simulink model "GravitationalBattery"  (R2020b)
settings: Solver=VariableStepAuto  StartTime=0.0  StopTime=1000000  RelTol=1e-9  AbsTol=1e-9
model workspace (MAT data in the model file):
  Sig = Simulink.Signal
  Sig.DataType = 'auto'
  Sig.Dimensions = -1
  Sig.DimensionsMode = 'auto'
  Sig.Complexity = 'auto'
  Sig.SampleTime = -1
  Sig.SamplingMode = 'auto'
  Sig1 = Simulink.Signal
  Sig1.DataType = 'auto'
  Sig1.Dimensions = -1
  Sig1.DimensionsMode = 'auto'
  Sig1.Complexity = 'auto'
  Sig1.SampleTime = -1
  Sig1.SamplingMode = 'auto'
  Sig2 = Simulink.Signal
  Sig2.DataType = 'auto'
  Sig2.Dimensions = -1
  Sig2.DimensionsMode = 'auto'
  Sig2.Complexity = 'auto'
  Sig2.SampleTime = -1
  Sig2.SamplingMode = 'auto'
  earth_gravitational_acceleration = Simulink.Parameter
  earth_gravitational_acceleration.Value = -9.806
  earth_gravitational_acceleration.Description = 'https://en.wikipedia.org/wiki/Standard_gravity'
  earth_gravitational_acceleration.DataType = 'double'
  earth_gravitational_acceleration.DocUnits = 'm^2/s'
  earth_gravitational_acceleration.Dimensions = [1 1]
  electrogenerator_coeff = Simulink.Parameter
  electrogenerator_coeff.DataType = 'double'
  electrogenerator_coeff.Min = 0
  electrogenerator_coeff.DocUnits = 'V/(rad/s)'
  electrogenerator_coeff.Dimensions = [0 0]
  gear_box_ration = Simulink.Parameter
  gear_box_ration.Value = 1
  gear_box_ration.Description = 'Gear box ration'
  gear_box_ration.DataType = 'double'
  gear_box_ration.Min = 0
  gear_box_ration.Dimensions = [1 1]
  initial_mass_height = Simulink.Parameter
  initial_mass_height.Value = 10000
  initial_mass_height.Description = 'https://en.wikipedia.org/wiki/Distance'
  initial_mass_height.DataType = 'double'
  initial_mass_height.Min = 0
  initial_mass_height.DocUnits = 'm'
  initial_mass_height.Dimensions = [1 1]
  resistance_value = Simulink.Parameter
  resistance_value.Value = 1
  resistance_value.Description = 'https://en.wikipedia.org/wiki/Electrical_resistance_and_conductance'
  resistance_value.DataType = 'double'
  resistance_value.Min = 0
  resistance_value.DocUnits = 'Ohm'
  resistance_value.Dimensions = [1 1]
  weight_mass = Simulink.Parameter
  weight_mass.Value = 1
  weight_mass.Description = 'https://en.wikipedia.org/wiki/Mass'
  weight_mass.DataType = 'double'
  weight_mass.Min = 0
  weight_mass.DocUnits = 'kg'
  weight_mass.Dimensions = [1 1]
  wheel_and_axel_radius = Simulink.Parameter
  wheel_and_axel_radius.Value = 1
  wheel_and_axel_radius.Description = 'Radius of perfect wheel and axel mechanism'
  wheel_and_axel_radius.DataType = 'double'
  wheel_and_axel_radius.Min = 0
  wheel_and_axel_radius.DocUnits = 'm'
  wheel_and_axel_radius.Dimensions = [1 1]
libraries: fl_lib x15, nesl_utility x9, simulink x1, sdl_lib x1
Description:
  | https://en.wikipedia.org/wiki/Gravity_battery
settings Model: OrderedModelArguments=off  Creator=ofcra  LastModifiedBy=ofcra
settings SolverCC: InitialStep=1

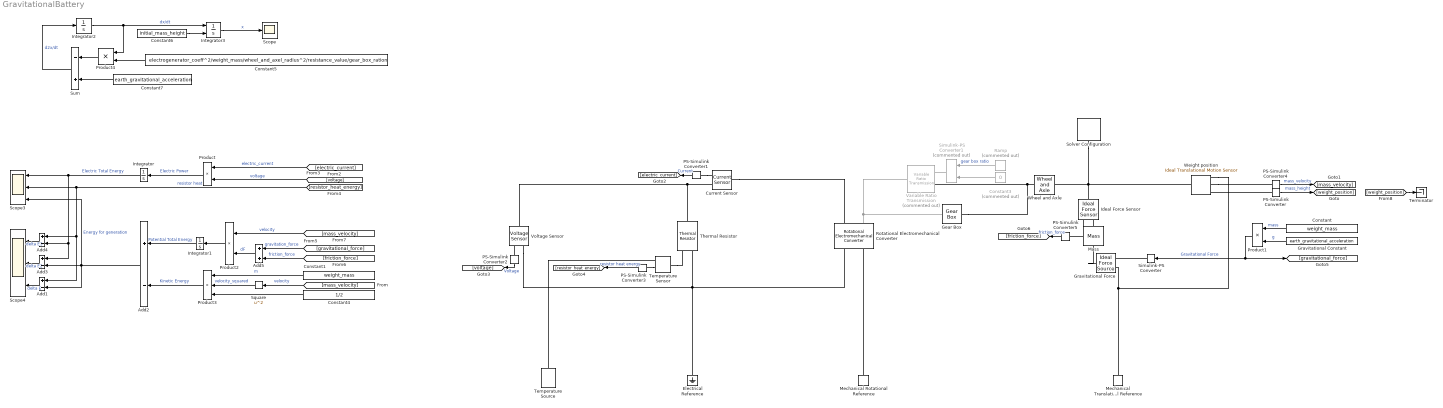
== system GravitationalBattery ==
  Add{1..4} (4 alike) : Sum  Inputs=+-
  Add5 : Sum
  Constant : Constant  Value=weight_mass
  Constant1 : Constant  Value=weight_mass
  Constant3 : Constant  Commented=on  Value=0
  Constant4 : Constant  Value=1/2
  Constant5 : Constant  Value=electrogenerator_coeff^2/weight_mass/wheel_and_axel_radius^2/resistance_value/gear_box_ration
  Constant6 : Constant  Value=initial_mass_height
  Constant7 : Constant  Value=earth_gravitational_acceleration
  Current Sensor : fl_lib/Electrical/Electrical Sensors/Current Sensor
  Electrical Reference : fl_lib/Electrical/Electrical Elements/Electrical Reference
  Gear Box : fl_lib/Mechanical/Mechanisms/Gear Box  ratio=gear_box_ration  t_in_specify=off  t_in_priority=None  t_in=0 N*m  t_in_nominal_specify=off  t_in_nominal_unit=N*m  t_in_nominal_value=1  t_out_specify=off  t_out_priority=None  t_out=0 N*m  t_out_nominal_specify=off  t_out_nominal_unit=N*m  t_out_nominal_value=1
  Gravitational Constant : Constant  Value=earth_gravitational_acceleration
  Gravitational Force : fl_lib/Mechanical/Mechanical Sources/Ideal Force Source
  Ideal Force Sensor : fl_lib/Mechanical/Mechanical Sensors/Ideal Force Sensor
  Integrator : Integrator
  Integrator1 : Integrator
  Integrator2 : Integrator
  Integrator3 : Integrator  InitialConditionSource=external
  Mass : fl_lib/Mechanical/Translational Elements/Mass  mass=weight_mass kg  num_ports=foundation.enum.numPorts2.two  v_specify=off  v_priority=High  v=0 m/s  v_nominal_specify=off  v_nominal_unit=m/s  v_nominal_value=1  f_specify=off  f_priority=None  f=0 N  f_nominal_specify=off  f_nominal_unit=N  f_nominal_value=1
      settings: InternalSimscapePortConfiguration="{\"Bottom\":[],\"Left\":[{\"id\":\"M\",\"label\":\"\",\"type\":\"foundation.mechanical.translational.translational\"}],\"Right\":[{\"id\":\"N\",\"label\":\"\",\"type\":\"foundation.mechanical.translational.translational\"}],\"Top\":[]}"
  Mechanical Rotational Reference : fl_lib/Mechanical/Rotational Elements/Mechanical Rotational Reference
  Mechanical Translational Reference : fl_lib/Mechanical/Translational Elements/Mechanical Translational Reference
  PS-Simulink Converter{,1..5} (6 alike) : nesl_utility/PS-Simulink Converter  PhysicalDomain=network_engine_domain  SubClassName=ps_output  LeftPortType=input  RightPortType=output  PseudoPeriodic=off  Frequencies=[]  Unit=inherit  AffineConversion=off
  Product{,1..2,4} (4 alike) : Product
  Product3 : Product  Inputs=3
  Ramp : simulink/Sources/Ramp  Commented=on  slope=0  start=0  InitialOutput=0.1
  Rotational Electromechanical Converter : fl_lib/Electrical/Electrical Elements/Rotational Electromechanical Converter  K=electrogenerator_coeff V/(rad/s)  i_specify=off  i_priority=None  i=0 A  i_nominal_specify=off  i_nominal_unit=A  i_nominal_value=1  v_specify=off  v_priority=None  v=0 V  v_nominal_specify=off  v_nominal_unit=V  v_nominal_value=1  t_specify=off  t_priority=None  t=0 N*m  t_nominal_specify=off  t_nominal_unit=N*m  t_nominal_value=1  w_specify=off  w_priority=None  w=0 rad/s  w_nominal_specify=off  w_nominal_unit=rad/s  w_nominal_value=1
  Scope : Scope
  Scope3 : Scope  NumInputPorts=3
  Scope4 : Scope  NumInputPorts=3
  Simulink-PS Converter : nesl_utility/Simulink-PS Converter  PhysicalDomain=network_engine_domain  SubClassName=ps_input  LeftPortType=input  RightPortType=output  PseudoPeriodic=off  Frequencies=[]  NoiseDistribution=none  NoiseParameters=[]  Unit=1  AffineConversion=off  FilteringAndDerivatives=provide  SimscapeFilterOrder=1  InputFilterTimeConstant=0.001  UdotUserProvided=0
  Simulink-PS Converter1 : nesl_utility/Simulink-PS Converter  Commented=on  PhysicalDomain=network_engine_domain  SubClassName=ps_input  LeftPortType=input  RightPortType=output  PseudoPeriodic=off  Frequencies=[]  NoiseDistribution=none  NoiseParameters=[]  Unit=1  AffineConversion=off  FilteringAndDerivatives=provide  SimscapeFilterOrder=1  InputFilterTimeConstant=0.001  UdotUserProvided=1
  Solver Configuration : nesl_utility/Solver Configuration  PhysicalDomain=network_engine_domain  SubClassName=solver  LeftPortType=input  RightPortType=generic  Tones=[]  Harmonics=[]  SimulateNoise=off  Profile=off  UseLocalSampling=off  EnableSwitchedLinearOptims=on  FrequencyDomain=off  UseCCode=off  RelTol=0.001  AbsTol=1e-06  MinStep=1e-09  ToWorkspace=off  RevertToSquareIcSolve=off  NumHomotopyIterations=100  PhasorMode=off  PhasorModeNumHarmonics=1  DoDC=off  ResidualTolerance=1e-09  UseLocalSolver=off  LocalSolverChoice=NE_BACKWARD_EULER_ADVANCER  LocalSolverSampleTime=0.001  DoFixedCost=off  MaxNonlinIter=3  MaxModeIter=2  ComputeImpulses=off  ImpulseIterations=2  LinearAlgebra=auto  EquationFormulation=NE_TIME_EF  DelaysMemoryBudget=1024  AutomaticFiltering=on  FilteringTimeConstant=0.001  PartitionStorageMethod=AS_NEEDED  PartitionMemoryBudget=1024  PartitionMethod=ROBUST
  Square : Math  Operator=square  SaturateOnIntegerOverflow=on
  Sum : Sum  Inputs=-+
  Temperature Sensor : fl_lib/Thermal/Thermal Sensors/Temperature Sensor
  Temperature Source : fl_lib/Thermal/Thermal Sources/Temperature Source  temperature=293.15 K
  Terminator : Terminator
  Thermal Resistor : fl_lib/Electrical/Electrical Elements/Thermal Resistor  R0=resistance_value Ohm  T0=293.15 K  alpha=0 1/K  tc=1 s  K_d=1 W/K  T_specify=on  T_priority=High  T=293.15 K  T_nominal_specify=off  T_nominal_unit=K  T_nominal_value=1
      settings: SourceProductBaseCode=SS  InternalSimscapePortConfiguration="{\"Bottom\":[],\"Left\":[{\"id\":\"H\",\"label\":\"H\",\"type\":\"foundation.thermal.thermal\"},{\"id\":\"p\",\"label\":\"+\",\"type\":\"foundation.electrical.electrical\"}],\"Right\":[{\"id\":\"n\",\"label\":\"-\",\"type\":\"foundation.electrical.electrical\"}],\"Top\":[]}"
  Variable Ratio Transmission : sdl_lib/Couplings & Drives/Variable Ratio Transmission  Commented=on  rotation_direction=1  kp=0.01 N*m/rad  kv=0.05 N*m/(rad/s)  initial_torque=0 N*m  losses_model=1  efficiency=0.9  mu_visc=[0, 0] N*m/(rad/s)  w_thr=0.01 rad/s  R_specify=off  R_priority=None  R=1  R_nominal_specify=off  R_nominal_unit=1  R_nominal_value=1
      settings: SourceProductBaseCode=LD  InternalSimscapePortConfiguration="{\"Bottom\":[],\"Left\":[{\"id\":\"ratio\",\"label\":\"r\",\"type\":\"input\"},{\"id\":\"B\",\"label\":\"B\",\"type\":\"foundation.mechanical.rotational.rotational\"}],\"Right\":[{\"id\":\"F\",\"label\":\"F\",\"type\":\"foundation.mechanical.rotational.rotational\"}],\"Top\":[]}"
  Voltage Sensor : fl_lib/Electrical/Electrical Sensors/Voltage Sensor
  Weight position : fl_lib/Mechanical/Mechanical Sensors/Ideal Translational Motion Sensor  offset=initial_mass_height m
  Wheel and Axle : fl_lib/Mechanical/Mechanisms/Wheel and Axle  R=wheel_and_axel_radius m  or=2  t_specify=off  t_priority=None  t=0 N*m  t_nominal_specify=off  t_nominal_unit=N*m  t_nominal_value=1  f_specify=off  f_priority=None  f=0 N  f_nominal_specify=off  f_nominal_unit=N  f_nominal_value=1
  wires:
  PS-Simulink Converter1/1 -> [electric_current]  "Current"
  Product/1 -> Integrator/1  "Electric Power"
  Ramp/1 -> Simulink-PS Converter1/1  "gear box ratio"
  Product1/1 -> [gravitational_force], Simulink-PS Converter/1  "Gravitational Force"
  Constant/1 -> Product1/1  "mass"
  Gravitational Constant/1 -> Product1/2  "g"
  Integrator/1 -> Add3/1, Add4/2, Scope3/1  "Electric Total Energy"
  Constant1/1 -> Product3/1  "m"
  Add1/1 -> Scope4/3  "delta E"
  Constant3/1 -> Simulink-PS Converter1/2
  Square/1 -> Product3/2  "velocity_squared"
  PS-Simulink Converter4/1 -> [mass_velocity]  "mass_velocity"
  Product3/1 -> Add2/2  "Kinetic Energy"
  Product2/1 -> Integrator1/1
  Add2/1 -> Add1/2, Add3/2, Scope3/3  "Energy for generation"
  Constant4/1 -> Product3/3
  Add3/1 -> Scope4/2  "delta E2"
  PS-Simulink Converter/1 -> [weight_position]  "mass_height"
  [mass_velocity] -> Square/1  "velocity"
  [electric_current] -> Product/1  "electric_current"
  [voltage] -> Product/2  "voltage"
  PS-Simulink Converter2/1 -> [voltage]  "Voltage"
  PS-Simulink Converter3/1 -> [resistor_heat_energy]  "resistor heat energy"
  [resistor_heat_energy] -> Add1/1, Add4/1, Scope3/2  "resistor heat"
  Add4/1 -> Scope4/1  "delta E3"
  PS-Simulink Converter5/1 -> [friction_force]  "friction_force"
  [gravitational_force] -> Add5/1  "gravitation_force"
  [friction_force] -> Add5/2  "friction_force"
  Add5/1 -> Product2/2  "dF"
  [mass_velocity] -> Product2/1  "velocity"
  Integrator1/1 -> Add2/1  "Potential Total Energy"
  Sum/1 -> Integrator2/1  "d2x/dt"
  Integrator2/1 -> Integrator3/1, Product4/1  "dx/dt"
  Integrator3/1 -> Scope/1  "x"
  Constant5/1 -> Product4/2
  Product4/1 -> Sum/1
  Constant6/1 -> Integrator3/2
  Constant7/1 -> Sum/2
  [weight_position] -> Terminator/1
  connections:
  Solver Configuration/RConn1 -- Ideal Force Sensor/LConn1 -- Weight position/LConn1 -- Wheel and Axle/RConn1
  Mechanical Translational Reference/LConn1 -- Weight position/RConn1 -- Gravitational Force/RConn2
  PS-Simulink Converter/LConn1 -- Weight position/RConn3
  Mechanical Rotational Reference/LConn1 -- Rotational Electromechanical Converter/RConn2
  Voltage Sensor/RConn2 -- Thermal Resistor/LConn2 -- Rotational Electromechanical Converter/RConn1 -- Electrical Reference/LConn1
  Voltage Sensor/LConn1 -- Thermal Resistor/RConn1 -- Current Sensor/RConn2
  PS-Simulink Converter1/LConn1 -- Current Sensor/RConn1
  PS-Simulink Converter2/LConn1 -- Voltage Sensor/RConn1
  Weight position/RConn2 -- PS-Simulink Converter4/LConn1
  Gravitational Force/LConn1 -- Mass/RConn1
  Simulink-PS Converter/RConn1 -- Gravitational Force/RConn1
  Simulink-PS Converter1/RConn1 -- Variable Ratio Transmission/LConn1
  Wheel and Axle/LConn1 -- Gear Box/LConn1 -- Variable Ratio Transmission/LConn2
  Variable Ratio Transmission/RConn1 -- Rotational Electromechanical Converter/LConn2 -- Gear Box/RConn1
  Temperature Sensor/LConn1 -- Thermal Resistor/LConn1
  Temperature Source/LConn1 -- Temperature Sensor/RConn1
  PS-Simulink Converter3/LConn1 -- Temperature Sensor/RConn2
  Current Sensor/LConn1 -- Rotational Electromechanical Converter/LConn1
  Ideal Force Sensor/RConn2 -- PS-Simulink Converter5/LConn1
  Mass/LConn1 -- Ideal Force Sensor/RConn1
